simulink model "shipController"  (Simulink 8.5)
settings: Solver=ode45  StartTime=0.0  StopTime=1500  RelTol=1e-3
values from neighbouring files (symbols this model uses):
  Kpd = 0.749    [vanLoan.m]
  Td = 87.14    [vanLoan.m]
  Tf = 8.391    [vanLoan.m]
  Ts = 1/fs    (= 0.1)    [Copy_of_Kalman.m]    (also in initKalman.m; vanLoan.m)
libraries: simulink x2
settings Model: Creator=markh  LastModifiedBy=jljoberg
settings DataIOCC: SignalLoggingName=sigsOut
settings OptimizationCC: ExpressionDepthLimit=128  InitFltsAndDblsToZero=on
settings DebuggingCC: SaveWithParameterizedLinksMsg=none  SignalResolutionControl=TryResolveAllWithWarning  MultiTaskDSMMsg=warning  MultiTaskCondExecSysMsg=none  FcnCallInpInsideContextMsg=UseLocalSettings
settings HardwareCC: TargetUnknown=on
settings GRTTargetCC: TargetFcnLib=ansi_tfl_tmw.mat

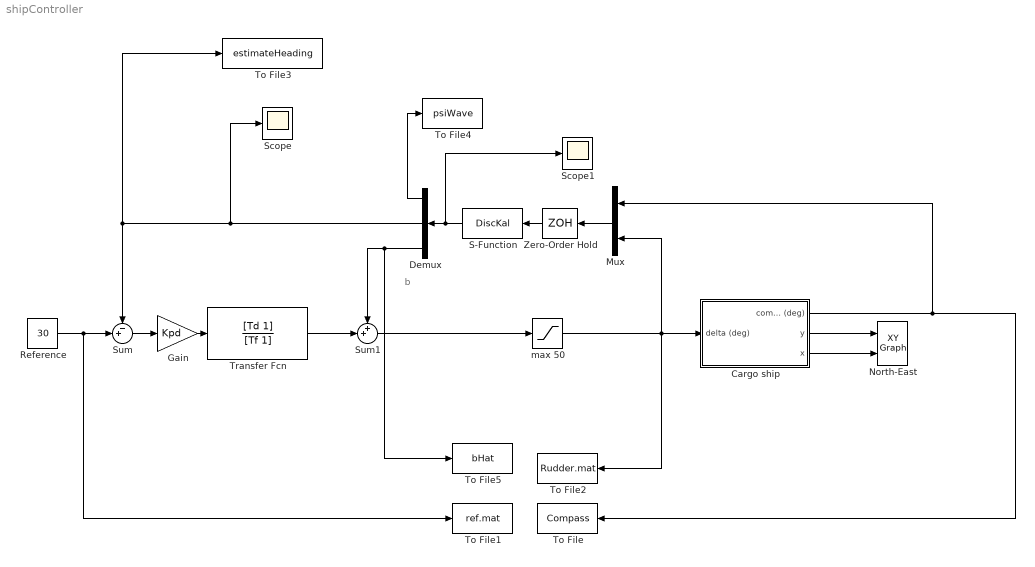
== system shipController ==
  note: b
  Cargo ship : Subsystem  mask(Simple shipmodel for a cargo ship){noise=on, current=on, logic=on}
      mask prompts: noise "measurement noise"; logic "waves"
      mask help:
      | Measurement noise:
      | 	checked = noise on
      | 	unchecked = noise off
      |
      | Current:
      | 	checked = current on
      | 	unchecked = current off
      |
      | Waves:
      | 	checked = waves on
      | 	unchecked = waves off
      |
      | Author: Jørgen Spjøtvold, 9/10-2003
      | TTK 4115 Linear system theory.
      | Modified by Jostein Bakkeheim 26/10-2006
  Demux : Demux  Outputs=3
  Gain : Gain  Gain=Kpd
  Mux : Mux  Inputs=2
  North-East : simulink/Sinks/XY Graph  xmin=-5000  xmax=5000  ymin=-5000  ymax=5000  st=-1
  Reference : Constant  Value=30
  S-Function : S-Function  FunctionName=DiscKal  Parameters=data
  Scope : Scope
      settings: YMin=17.5  YMax=26
  Scope1 : Scope
      settings: YMin=-2.5  YMax=30
  Sum : Sum  Inputs=-+|
  Sum1 : Sum  Inputs=++|
  To File : ToFile  Filename=Compass  MatrixName=Compass
  To File1 : ToFile  Filename=ref.mat  MatrixName=ref
  To File2 : ToFile  Filename=Rudder.mat  MatrixName=Rudder
  To File3 : ToFile  Filename=estimateHeading  MatrixName=estimateHeading
  To File4 : ToFile  Filename=psiWave  MatrixName=psiWave
  To File5 : ToFile  Filename=bHat  MatrixName=bHat
  Transfer Fcn : TransferFcn  Numerator=[Td 1]  Denominator=[Tf 1]
  Zero-Order Hold : ZeroOrderHold  SampleTime=Ts
  max 50 : Saturate  UpperLimit=50  LowerLimit=-50
  wires:
  Cargo ship/3(x) -> North-East/2
  Cargo ship/2(y) -> North-East/1
  Cargo ship/1(compass (deg)) -> Mux/1, To File/1
  Gain/1 -> Transfer Fcn/1
  Reference/1 -> Sum/2, To File1/1
  Mux/1 -> Zero-Order Hold/1
  Zero-Order Hold/1 -> S-Function/1
  Sum/1 -> Gain/1
  Sum1/1 -> max 50/1
  max 50/1 -> To File2/1, Cargo ship/1(delta (deg)), Mux/2
  Transfer Fcn/1 -> Sum1/2
  Demux/3 -> To File5/1, Sum1/1
  Demux/2 -> Scope/1, Sum/1, To File3/1
  Demux/1 -> To File4/1
  S-Function/1 -> Scope1/1, Demux/1

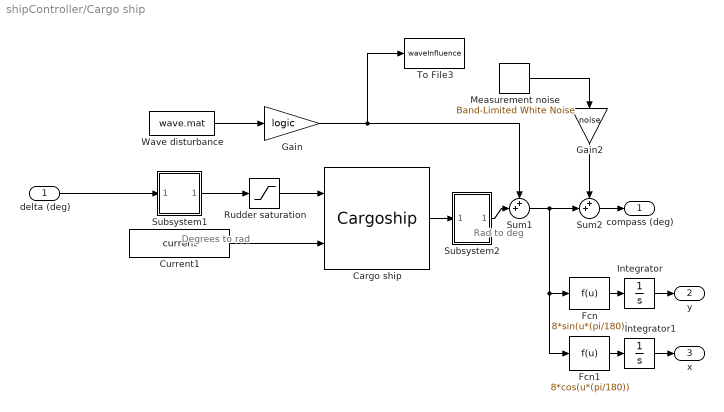
== system shipController/Cargo ship ==
  note: Degrees to rad
  note: Rad to deg
  delta (deg) : Inport
  Cargo ship : S-Function  FunctionName=Cargoship  mask(Cargo ship){}
      mask help:
      | S-function which simulates a cargo ship.
      |
      | Author: Jørgen Spjøtvold
      | 20.10-2003
      | Modified by Jostein Bakkeheim 27.10.2006
  Current1 : Constant  Value=current
  Fcn : Fcn  Expr=8*sin(u*(pi/180))
  Fcn1 : Fcn  Expr=8*cos(u*(pi/180))
  Gain : Gain  Gain=logic  SaturateOnIntegerOverflow=on  OutDataTypeStr=Inherit: Same as input  ParamDataTypeStr=Inherit: Same as input
  Gain2 : Gain  Gain=noise  SaturateOnIntegerOverflow=on  OutDataTypeStr=Inherit: Same as input  ParamDataTypeStr=Inherit: Same as input
  Integrator : Integrator
  Integrator1 : Integrator
  Measurement noise : simulink/Sources/Band-Limited White Noise  Cov=[0.001]  Ts=.5  seed=[23341]
  Rudder saturation : Saturate  UpperLimit=45*(pi/180)  LowerLimit=-45*(pi/180)
  Subsystem1 : Subsystem  mask(degrees to radians){}
      mask help: Converts degrees to radians
      mask Display: fprintf('D2R');
  Subsystem2 : Subsystem  mask(radians to degrees){}
      mask help: Converts radians to degrees
      mask Display: fprintf('R2D');
  Sum1 : Sum  Inputs=++|  SaturateOnIntegerOverflow=on
  Sum2 : Sum  Inputs=++|  SaturateOnIntegerOverflow=on
  To File3 : ToFile  Filename=waveInfluence  MatrixName=waveInfluence
  Wave disturbance : FromFile  FileName=wave.mat  SampleTime=0
  compass (deg) : Outport
  y : Outport  Port=2
  x : Outport  Port=3
  wires:
  delta (deg)/1 -> Subsystem1/1(In1)
  Fcn/1 -> Integrator/1
  Integrator/1 -> y/1
  Fcn1/1 -> Integrator1/1
  Integrator1/1 -> x/1
  Wave disturbance/1 -> Gain/1
  Subsystem2/1(Out1) -> Sum1/2
  Gain/1 -> To File3/1, Sum1/1
  Sum1/1 -> Fcn/1, Fcn1/1, Sum2/2
  Cargo ship/1 -> Subsystem2/1(In1)
  Subsystem1/1(Out1) -> Rudder saturation/1
  Rudder saturation/1 -> Cargo ship/1
  Sum2/1 -> compass (deg)/1
  Measurement noise/1 -> Gain2/1
  Gain2/1 -> Sum2/1
  Current1/1 -> Cargo ship/2

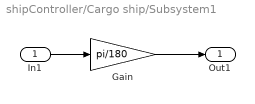
== system shipController/Cargo ship/Subsystem1 ==
  In1 : Inport
  Gain : Gain  Gain=pi/180  SaturateOnIntegerOverflow=on  OutDataTypeStr=Inherit: Same as input  ParamDataTypeStr=Inherit: Same as input
  Out1 : Outport
  wires:
  Gain/1 -> Out1/1
  In1/1 -> Gain/1

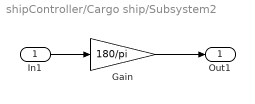
== system shipController/Cargo ship/Subsystem2 ==
  In1 : Inport
  Gain : Gain  Gain=180/pi  SaturateOnIntegerOverflow=on  OutDataTypeStr=Inherit: Same as input  ParamDataTypeStr=Inherit: Same as input
  Out1 : Outport
  wires:
  Gain/1 -> Out1/1
  In1/1 -> Gain/1
